simulink model "Control_Unit_Software_Case3"  (R2018b)
settings: Solver=FixedStepAuto  StartTime=0.0  StopTime=2  RelTol=1e-3
values from neighbouring files (symbols this model uses):
  A = [-(bm*(n^2) + bg)/(Jm*(n^2) + Jg) Kt*n/(Jm*(n^2) + Jg) ... (first row only)    [acceptatieTestScript.m]
  B = [0 ... (first row only)    [acceptatieTestScript.m]
  C = [1 0]    [acceptatieTestScript.m]
  D = [0]    [acceptatieTestScript.m]
  Kdi = dlqr(Ad,Bd,Q,R)    [acceptatieTestScript.m]
  n = 16.5    [acceptatieTestScript.m]
  Tsc = 1/20000    (= 5e-05)    [acceptatieTestScript.m]
undefined symbols (not defined in the file or in its folder): DiscIntNeverNeededParam, sigbuilder_block
libraries: dspswit3 x29, simulink x14, powerlib_meascontrol x6, dspsigops x4, pePwmGenerator x4, peLuenbergerObserver x2, peGeneralControl x1
(part 1 of 2)
settings Model: Creator=Roberto  LastModifiedBy=Roberto

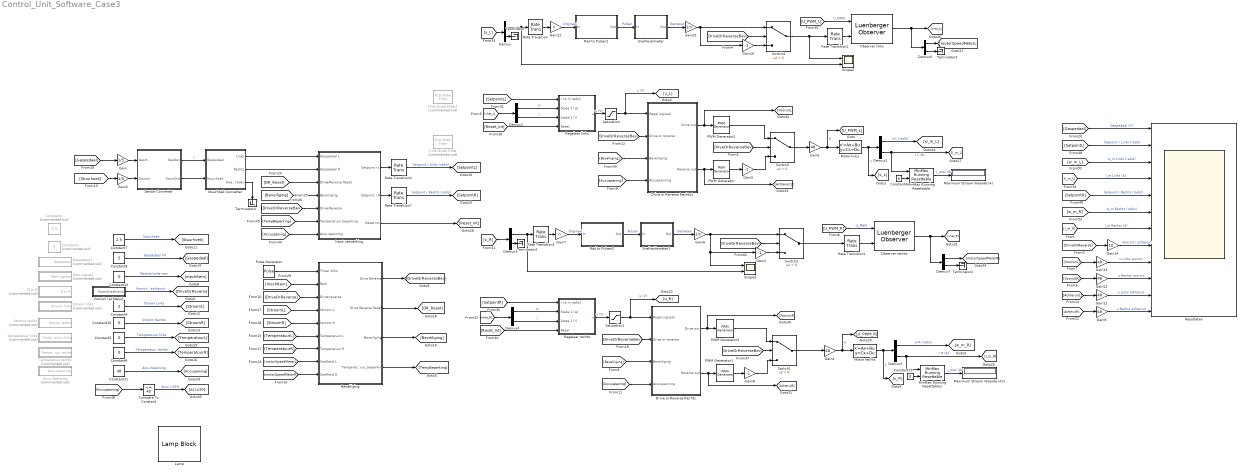
== system Control_Unit_Software_Case3 ==
  Accu Spanning : Subsystem  Tag=STV Subsys  Commented=on  LoadFcn=sigbuilder_block('load');  StartFcn=sigbuilder_block('start');  StopFcn=sigbuilder_block('stop');  ClipboardFcn=sigbuilder_block('clipboard');  mask(Sigbuilder block){tuvar=[0:10]}
      mask help: Simulink:masks:SigbuilderBlock_MD
      mask init:
      | if ~strcmp(get_param(bdroot(gcbh),'SimulationStatus'),'stopped') tuvar = sigbuilder_block('maskInit'); end
      settings: CopyFcn=sigbuilder_block('copy');  DeleteFcn=sigbuilder_block('delete');  ModelCloseFcn=sigbuilder_block('modelClose');  PreSaveFcn=sigbuilder_block('preSave');  PauseFcn=sigbuilder_block('pause');  ContinueFcn=sigbuilder_block('continue');  NameChangeFcn=sigbuilder_block('namechange');  OpenFcn=sigbuilder_block('open',[341.25 138 550.5 359.25 ]);  CloseFcn=sigbuilder_block('close');
      mask Display: plot(0, 0, 100, 100,[2, 2, 32, 32, 2], [68, 8, 8, 68, 68],[32, 2], [38, 38], [32, 19, 2],[53, 60, 44], [32, 17, 17, 2],[16, 16, 31, 31]);txt = getActiveGroup(gcbh);text(2, 100, txt,'verticalAlignment', 'top');
  Beveiliging : Subsystem
  Compare To Constant : simulink/Logic and Bit Operations/Compare To Constant  relop=<=  const=40  OutDataTypeStr=boolean
  Constant{4..6,9..10,13,15} (7 alike) : Constant  Value=0
  Constant11 : Constant  Value=48
  Constant2 : Constant  Commented=on  Value=2.5
  Constant3 : Constant  Commented=on  Value=5
  Constant7 : Constant  Value=2.5
  Constant8 : Constant  Value=5
  D or R : Subsystem  Tag=STV Subsys  Commented=on  LoadFcn=sigbuilder_block('load');  StartFcn=sigbuilder_block('start');  StopFcn=sigbuilder_block('stop');  ClipboardFcn=sigbuilder_block('clipboard');  mask(Sigbuilder block){tuvar=[0:10]}
      mask help: Simulink:masks:SigbuilderBlock_MD
      mask init:
      | if ~strcmp(get_param(bdroot(gcbh),'SimulationStatus'),'stopped') tuvar = sigbuilder_block('maskInit'); end
      settings: CopyFcn=sigbuilder_block('copy');  DeleteFcn=sigbuilder_block('delete');  ModelCloseFcn=sigbuilder_block('modelClose');  PreSaveFcn=sigbuilder_block('preSave');  PauseFcn=sigbuilder_block('pause');  ContinueFcn=sigbuilder_block('continue');  NameChangeFcn=sigbuilder_block('namechange');  OpenFcn=sigbuilder_block('open',[437.6 153 550.4 359.25 ]);  CloseFcn=sigbuilder_block('close');
      mask Display: plot(0, 0, 100, 100,[2, 2, 32, 32, 2], [68, 8, 8, 68, 68],[32, 2], [38, 38], [32, 19, 2],[53, 60, 44], [32, 17, 17, 2],[16, 16, 31, 31]);txt = getActiveGroup(gcbh);text(2, 100, txt,'verticalAlignment', 'top');
  Demux{,1..7} (8 alike) : Demux  Outputs=2
  Drive or Reverse Rechts : Subsystem
  Drive or Reverse Rechts1 : Subsystem
  First-Order Filter : powerlib_meascontrol/Filters/First-Order Filter  Commented=on  FilterType=Lowpass  Tc=1.2  Ts=Tsc  Initialize=on  Vac_Init=[0, 0, 60]  Vdc_Init=0  PlotResponse=off  FreqRange="[0,  200,  1]"
      settings: SourceProductName=Simscape Power Systems
  First-Order Filter1 : powerlib_meascontrol/Filters/First-Order Filter  Commented=on  FilterType=Lowpass  Tc=1.2  Ts=Tsc  Initialize=on  Vac_Init=[0, 0, 60]  Vdc_Init=0  PlotResponse=off  FreqRange="[0,  200,  1]"
      settings: SourceProductName=Simscape Power Systems
  Gain : Gain  Gain=1/5
  Gain{1,4,9,11..13} (6 alike) : Gain  Gain=48
  Gain{2,5,8,10} (4 alike) : Gain  Gain=-1
  Gain14 : Gain  Gain=10
  Gain21 : Gain  Gain=1/n
  Gain22 : Gain  Gain=n
  Gain3 : Gain  Gain=1/5
  Gain6 : Gain  Gain=1/n
  Gain7 : Gain  Gain=n
  Gaspedaal1 : Subsystem  Tag=STV Subsys  Commented=on  LoadFcn=sigbuilder_block('load');  StartFcn=sigbuilder_block('start');  StopFcn=sigbuilder_block('stop');  ClipboardFcn=sigbuilder_block('clipboard');  mask(Sigbuilder block){tuvar=[0:10]}
      mask help: Simulink:masks:SigbuilderBlock_MD
      mask init:
      | if ~strcmp(get_param(bdroot(gcbh),'SimulationStatus'),'stopped') tuvar = sigbuilder_block('maskInit'); end
      settings: CopyFcn=sigbuilder_block('copy');  DeleteFcn=sigbuilder_block('delete');  ModelCloseFcn=sigbuilder_block('modelClose');  PreSaveFcn=sigbuilder_block('preSave');  PauseFcn=sigbuilder_block('pause');  ContinueFcn=sigbuilder_block('continue');  NameChangeFcn=sigbuilder_block('namechange');  OpenFcn=sigbuilder_block('open',[468 234 550.5 278.25 ]);  CloseFcn=sigbuilder_block('close');
      mask Display: plot(0, 0, 100, 100,[2, 2, 32, 32, 2], [68, 8, 8, 68, 68],[32, 2], [38, 38], [32, 19, 2],[53, 60, 44], [32, 17, 17, 2],[16, 16, 31, 31]);txt = getActiveGroup(gcbh);text(2, 100, txt,'verticalAlignment', 'top');
  Input verwerking : Subsystem
  Lamp : LampBlock  WebBlockId=979
  Maximum Stroom Waarde (A) : Display
  Maximum Stroom Waarde (A)1 : Display
  MinMax Running Resettable : simulink/Math Operations/MinMax Running Resettable  Function=max  vinit=0.0
  MinMax Running Resettable1 : simulink/Math Operations/MinMax Running Resettable  Function=max  vinit=0.0
  Motor links : StateSpace  A=A  B=B  C=eye(2)  D=[0; 0]  InitialCondition=0
  Motor rechts : StateSpace  A=A  B=B  C=eye(2)  D=[0; 0]  InitialCondition=0
  Observer links : peLuenbergerObserver/Luenberger Observer  StateSpaceType=Continuous-time  Ad=Adh  Bd=Bdh  Cd=C  Dd=0  A=A  B=B  C=C  D=D  ObserverDesign=Observer gain  Ld=L  DesiredEigenvalues=eigenVal  x0=[0 0]  Tsd=0.1  Ts=1e-6
  Observer rechts : peLuenbergerObserver/Luenberger Observer  StateSpaceType=Continuous-time  Ad=Adh  Bd=Bdh  Cd=C  Dd=0  A=A  B=B  C=C  D=D  ObserverDesign=Observer gain  Ld=L  DesiredEigenvalues=eigenVal  x0=[0 0]  Tsd=0.1  Ts=1e-6
  PWM Generator{,1..3} (4 alike) : pePwmGenerator/PWM Generator  CarrCount=Up  Tper=1/20000  Ts=1e-6
  Pulse Generator : DiscretePulseGenerator  SampleTime=1/2000
  Rad to Pulsen1 : Subsystem
  Rad to Pulsen2 : Subsystem
  Rate Transition : RateTransition  OutPortSampleTime=1/100000
  Rate Transition1 : RateTransition  OutPortSampleTime=1e-6
  Rate Transition2 : RateTransition  OutPortSampleTime=Tsc
  Rate Transition3 : RateTransition  OutPortSampleTime=1/100000
  Rate Transition4 : RateTransition  OutPortSampleTime=1e-6
  Rate Transition7 : RateTransition  OutPortSampleTime=Tsc
  Regelaar links : Subsystem
  Regelaar rechts : Subsystem
  Rem signaal : Subsystem  Tag=STV Subsys  Commented=on  LoadFcn=sigbuilder_block('load');  StartFcn=sigbuilder_block('start');  StopFcn=sigbuilder_block('stop');  ClipboardFcn=sigbuilder_block('clipboard');  mask(Sigbuilder block){tuvar=[0:10]}
      mask help: Simulink:masks:SigbuilderBlock_MD
      mask init:
      | if ~strcmp(get_param(bdroot(gcbh),'SimulationStatus'),'stopped') tuvar = sigbuilder_block('maskInit'); end
      settings: CopyFcn=sigbuilder_block('copy');  DeleteFcn=sigbuilder_block('delete');  ModelCloseFcn=sigbuilder_block('modelClose');  PreSaveFcn=sigbuilder_block('preSave');  PauseFcn=sigbuilder_block('pause');  ContinueFcn=sigbuilder_block('continue');  NameChangeFcn=sigbuilder_block('namechange');  OpenFcn=sigbuilder_block('open',[437.6 153 550.4 359.25 ]);  CloseFcn=sigbuilder_block('close');
      mask Display: plot(0, 0, 100, 100,[2, 2, 32, 32, 2], [68, 8, 8, 68, 68],[32, 2], [38, 38], [32, 19, 2],[53, 60, 44], [32, 17, 17, 2],[16, 16, 31, 31]);txt = getActiveGroup(gcbh);text(2, 100, txt,'verticalAlignment', 'top');
  Resultaten : Scope  NumInputPorts=12
  Saturation : Saturate  UpperLimit=60  LowerLimit=-60
  Saturation1 : Saturate  UpperLimit=60  LowerLimit=-60
  Scope3 : Scope  NumInputPorts=2
  Scope5 : Scope  NumInputPorts=2
  Sensor Converter : Subsystem
  Snelheidsmeter : Subsystem
  Snelheidsmeter1 : Subsystem
  Stroom links : Subsystem  Tag=STV Subsys  Commented=on  LoadFcn=sigbuilder_block('load');  StartFcn=sigbuilder_block('start');  StopFcn=sigbuilder_block('stop');  ClipboardFcn=sigbuilder_block('clipboard');  mask(Sigbuilder block){tuvar=[0:10]}
      mask help: Simulink:masks:SigbuilderBlock_MD
      mask init:
      | if ~strcmp(get_param(bdroot(gcbh),'SimulationStatus'),'stopped') tuvar = sigbuilder_block('maskInit'); end
      settings: CopyFcn=sigbuilder_block('copy');  DeleteFcn=sigbuilder_block('delete');  ModelCloseFcn=sigbuilder_block('modelClose');  PreSaveFcn=sigbuilder_block('preSave');  PauseFcn=sigbuilder_block('pause');  ContinueFcn=sigbuilder_block('continue');  NameChangeFcn=sigbuilder_block('namechange');  OpenFcn=sigbuilder_block('open',[437.6 153 550.4 359.25 ]);  CloseFcn=sigbuilder_block('close');
      mask Display: plot(0, 0, 100, 100,[2, 2, 32, 32, 2], [68, 8, 8, 68, 68],[32, 2], [38, 38], [32, 19, 2],[53, 60, 44], [32, 17, 17, 2],[16, 16, 31, 31]);txt = getActiveGroup(gcbh);text(2, 100, txt,'verticalAlignment', 'top');
  Stroom rechts : Subsystem  Tag=STV Subsys  Commented=on  LoadFcn=sigbuilder_block('load');  StartFcn=sigbuilder_block('start');  StopFcn=sigbuilder_block('stop');  ClipboardFcn=sigbuilder_block('clipboard');  mask(Sigbuilder block){tuvar=[0:10]}
      mask help: Simulink:masks:SigbuilderBlock_MD
      mask init:
      | if ~strcmp(get_param(bdroot(gcbh),'SimulationStatus'),'stopped') tuvar = sigbuilder_block('maskInit'); end
      settings: CopyFcn=sigbuilder_block('copy');  DeleteFcn=sigbuilder_block('delete');  ModelCloseFcn=sigbuilder_block('modelClose');  PreSaveFcn=sigbuilder_block('preSave');  PauseFcn=sigbuilder_block('pause');  ContinueFcn=sigbuilder_block('continue');  NameChangeFcn=sigbuilder_block('namechange');  OpenFcn=sigbuilder_block('open',[437.6 153 550.4 359.25 ]);  CloseFcn=sigbuilder_block('close');
      mask Display: plot(0, 0, 100, 100,[2, 2, 32, 32, 2], [68, 8, 8, 68, 68],[32, 2], [38, 38], [32, 19, 2],[53, 60, 44], [32, 17, 17, 2],[16, 16, 31, 31]);txt = getActiveGroup(gcbh);text(2, 100, txt,'verticalAlignment', 'top');
  Stuurhoek Converter : Subsystem
  Switch{1..4} (4 alike) : Switch  Criteria=u2 > Threshold
  Temperatuur links : Subsystem  Tag=STV Subsys  Commented=on  LoadFcn=sigbuilder_block('load');  StartFcn=sigbuilder_block('start');  StopFcn=sigbuilder_block('stop');  ClipboardFcn=sigbuilder_block('clipboard');  mask(Sigbuilder block){tuvar=[0:10]}
      mask help: Simulink:masks:SigbuilderBlock_MD
      mask init:
      | if ~strcmp(get_param(bdroot(gcbh),'SimulationStatus'),'stopped') tuvar = sigbuilder_block('maskInit'); end
      settings: CopyFcn=sigbuilder_block('copy');  DeleteFcn=sigbuilder_block('delete');  ModelCloseFcn=sigbuilder_block('modelClose');  PreSaveFcn=sigbuilder_block('preSave');  PauseFcn=sigbuilder_block('pause');  ContinueFcn=sigbuilder_block('continue');  NameChangeFcn=sigbuilder_block('namechange');  OpenFcn=sigbuilder_block('open',[437.6 153 550.4 359.25 ]);  CloseFcn=sigbuilder_block('close');
      mask Display: plot(0, 0, 100, 100,[2, 2, 32, 32, 2], [68, 8, 8, 68, 68],[32, 2], [38, 38], [32, 19, 2],[53, 60, 44], [32, 17, 17, 2],[16, 16, 31, 31]);txt = getActiveGroup(gcbh);text(2, 100, txt,'verticalAlignment', 'top');
  Temperatuur rechts : Subsystem  Tag=STV Subsys  Commented=on  LoadFcn=sigbuilder_block('load');  StartFcn=sigbuilder_block('start');  StopFcn=sigbuilder_block('stop');  ClipboardFcn=sigbuilder_block('clipboard');  mask(Sigbuilder block){tuvar=[0:10]}
      mask help: Simulink:masks:SigbuilderBlock_MD
      mask init:
      | if ~strcmp(get_param(bdroot(gcbh),'SimulationStatus'),'stopped') tuvar = sigbuilder_block('maskInit'); end
      settings: CopyFcn=sigbuilder_block('copy');  DeleteFcn=sigbuilder_block('delete');  ModelCloseFcn=sigbuilder_block('modelClose');  PreSaveFcn=sigbuilder_block('preSave');  PauseFcn=sigbuilder_block('pause');  ContinueFcn=sigbuilder_block('continue');  NameChangeFcn=sigbuilder_block('namechange');  OpenFcn=sigbuilder_block('open',[437.6 153 550.4 359.25 ]);  CloseFcn=sigbuilder_block('close');
      mask Display: plot(0, 0, 100, 100,[2, 2, 32, 32, 2], [68, 8, 8, 68, 68],[32, 2], [38, 38], [32, 19, 2],[53, 60, 44], [32, 17, 17, 2],[16, 16, 31, 31]);txt = getActiveGroup(gcbh);text(2, 100, txt,'verticalAlignment', 'top');
  Terminator{,1..4} (5 alike) : Terminator
  Vooruit / achteruit : Subsystem  Tag=STV Subsys  LoadFcn=sigbuilder_block('load');  StartFcn=sigbuilder_block('start');  StopFcn=sigbuilder_block('stop');  ClipboardFcn=sigbuilder_block('clipboard');  mask(Sigbuilder block){tuvar=[0:10]}
      mask help: Simulink:masks:SigbuilderBlock_MD
      mask init:
      | if ~strcmp(get_param(bdroot(gcbh),'SimulationStatus'),'stopped') tuvar = sigbuilder_block('maskInit'); end
      settings: CopyFcn=sigbuilder_block('copy');  DeleteFcn=sigbuilder_block('delete');  ModelCloseFcn=sigbuilder_block('modelClose');  PreSaveFcn=sigbuilder_block('preSave');  PauseFcn=sigbuilder_block('pause');  ContinueFcn=sigbuilder_block('continue');  NameChangeFcn=sigbuilder_block('namechange');  OpenFcn=sigbuilder_block('open',[468 255.75 550.5 237.75 ]);  CloseFcn=sigbuilder_block('close');
      mask Display: plot(0, 0, 100, 100,[2, 2, 32, 32, 2], [68, 8, 8, 68, 68],[32, 2], [38, 38], [32, 19, 2],[53, 60, 44], [32, 17, 17, 2],[16, 16, 31, 31]);txt = getActiveGroup(gcbh);text(2, 100, txt,'verticalAlignment', 'top');
  wires:
  Gain1/1 -> [U_PWM_L], Motor links/1  "U"
  Switch2/1 -> Gain1/1
  Demux1/2 -> Regelaar links/3(State 1 (I))  "I"
  Demux1/1 -> Regelaar links/2(State 1 (w))  "w"
  [Reset_Int] -> Regelaar links/4(Reset)
  [xhat_L] -> Demux1/1
  MinMax Running Resettable/1 -> Maximum Stroom Waarde (A)/1  "I_max (A)"
  Constant4/1 -> MinMax Running Resettable/2
  Demux2/2 -> [I_m_L], MinMax Running Resettable/1  "I L (A)"
  Demux2/1 -> [w_m_L]  "w L (rad/s)"
  Motor links/1 -> Demux2/1, [x_L]  "x"
  [U_PWM_L] -> Observer links/1  "U_PWM"
  Rad to Pulsen1/1(Out) -> Snelheidsmeter/1(In)  "Pulsen"
  Rate Transition1/1 -> Observer links/2
  Rate Transition/1 -> Gain22/1
  Snelheidsmeter/1(Out) -> Gain21/1  "Gemeten"
  Gain22/1 -> Rad to Pulsen1/1(In)  "Orgineel"
  Switch4/1 -> Rate Transition1/1, Scope5/1
  [x_L] -> Demux/1
  Demux/1 -> Scope5/2, Rate Transition/1
  Demux/2 -> Terminator/1
  Observer links/1 -> Demux6/1, [xhat_L]
  Beveiliging/1("Drive Reverse ") -> [DriveOrReverseBev]
  Gain/1 -> Sensor Converter/1(GasIn)
  Stuurhoek Converter/1(Links) -> Input verwerking/1(Gaspedaal L)
  Input verwerking/1(Setpoint r L) -> Rate Transition2/1
  Gain3/1 -> Sensor Converter/2(StuurIn)
  Input verwerking/3(Reset Int) -> [Reset_Int]
  Sensor Converter/2(StuurOut) -> Stuurhoek Converter/2(Stuurhoek)
  [DriveOrReverse] -> Beveiliging/3(Drive/reverse)
  [motorSpeedMeterR] -> Beveiliging/9(Snelheid R)
  [TemperatuurL] -> Beveiliging/6(Temperatuur L)
  [StroomR] -> Beveiliging/5(Stroom R)
  [StroomL] -> Beveiliging/4(Stroom L)
  Beveiliging/3(Beveiliging) -> [Beveiliging]
  [motorSpeedMeterL] -> Beveiliging/8(Snelheid L)
  Input verwerking/2(Setpoint r R) -> Rate Transition7/1
  Beveiliging/2(Drive Reverse Reset) -> [DR_Reset]
  [Stuurhoek] -> Gain3/1
  Stuurhoek Converter/2(Rechts) -> Input verwerking/2(Gaspedaal R)
  [mechRem] -> Beveiliging/2(Rem)
  [DR_Reset] -> Input verwerking/3(Drive/Reverse Reset)
  [Beveiliging] -> Input verwerking/4(Beveiliging)
  Pulse Generator/1 -> Beveiliging/1(Timer 1khz)
  [Gaspedaal] -> Gain/1
  [DriveOrReverseBev] -> Input verwerking/5(Drive/Reverse)
  Rate Transition7/1 -> [SetpointR]  "Setpoint r Rechts (rad/s)"
  Rate Transition2/1 -> [SetpointL]  "Setpoint r Links (rad/s)"
  [TemperatuurR] -> Beveiliging/7(Temperatuur R)
  Observer rechts/1 -> Demux7/1, [xhat_R]
  Demux5/1 -> [w_m_R]  "w R (rad/s)"
  Demux4/2 -> Regelaar rechts/3(State 1 (I))  "I"
  Rate Transition4/1 -> Observer rechts/2
  Gain7/1 -> Rad to Pulsen2/1(In)  "Orgineel"
  Switch1/1 -> Gain4/1
  [U_PWM_R] -> Observer rechts/1  "U_PWM"
  Snelheidsmeter1/1(Out) -> Gain6/1  "Gemeten"
  [Reset_Int] -> Regelaar rechts/4(Reset)
  [xhat_R] -> Demux4/1
  Demux3/1 -> Scope3/2, Rate Transition3/1
  MinMax Running Resettable1/1 -> Maximum Stroom Waarde (A)1/1  "I_max (A)"
  Demux5/2 -> [I_m_R], MinMax Running Resettable1/1  "I R (A)"
  [x_R] -> Demux3/1
  Motor rechts/1 -> [x_R], Demux5/1  "x"
  Rad to Pulsen2/1(Out) -> Snelheidsmeter1/1(In)  "Pulsen"
  Demux4/1 -> Regelaar rechts/2(State 1 (w))  "w"
  Constant15/1 -> MinMax Running Resettable1/2
  Gain4/1 -> [U_PWM_R], Motor rechts/1  "U"
  Demux3/2 -> Terminator2/1
  Rate Transition3/1 -> Gain7/1
  [SetpointL] -> Regelaar links/1(r (w in rad/s))
  [SetpointR] -> Regelaar rechts/1(r (w in rad/s))
  [Beveiliging] -> Drive or Reverse Rechts/3(Beveiliging)
  [DriveOrReverseBev] -> Switch1/2
  Drive or Reverse Rechts/1(Drive out) -> [VooruitR], PWM Generator3/1
  [Accuspaning] -> Drive or Reverse Rechts/4(Accuspanning)
  [DriveOrReverseBev] -> Drive or Reverse Rechts/2(Drive or reverse)
  Drive or Reverse Rechts/2(Reverse out) -> [AchteruitR], PWM Generator1/1
  Regelaar rechts/1(u) -> Saturation1/1  "u (V)"
  [Beveiliging] -> Drive or Reverse Rechts1/3(Beveiliging)
  [DriveOrReverseBev] -> Switch2/2
  Drive or Reverse Rechts1/1(Drive out) -> [VooruitL], PWM Generator2/1
  [Accuspaning] -> Drive or Reverse Rechts1/4(Accuspanning)
  [DriveOrReverseBev] -> Drive or Reverse Rechts1/2(Drive or reverse)
  Drive or Reverse Rechts1/2(Reverse out) -> [AchteruitL], PWM Generator/1
  Regelaar links/1(u) -> Saturation/1  "u (V)"
  Constant8/1 -> [Gaspedaal]  "Gaspedaal (V)"
  Constant13/1 -> [mechRem]  "Mechanische rem"
  Vooruit / achteruit/1(Vooruit/achteruit) -> [DriveOrReverse]  "Vooruit / achteruit"
  Constant9/1 -> [StroomL]  "Stroom Links"
  Constant6/1 -> [TemperatuurR]  "Temperatuur rechts"
  Constant7/1 -> [Stuurhoek]  "Stuurhoek"
  Constant10/1 -> [StroomR]  "Stroom Rechts"
  Constant5/1 -> [TemperatuurL]  "Temperatuur links"
  Constant11/1 -> [Accuspaning]  "Accu Spanning"
  Beveiliging/4(Temperatuur_beperking) -> [TempBeperking]
  [Accuspaning] -> Input verwerking/7(Accu spanning)
  [TempBeperking] -> Input verwerking/6(Temperatuur beperking)
  Gain6/1 -> Scope3/1, Gain2/1, Switch3/1
  [DriveOrReverseBev] -> Switch3/2
  Gain2/1 -> Switch3/3
  Switch3/1 -> Rate Transition4/1
  Gain21/1 -> Gain10/1, Switch4/1
  Gain10/1 -> Switch4/3
  [DriveOrReverseBev] -> Switch4/2
  Gain5/1 -> Switch2/3
  Gain8/1 -> Switch1/3
  PWM Generator/1 -> Gain5/1
  PWM Generator2/1 -> Switch2/1
  PWM Generator1/1 -> Gain8/1
  PWM Generator3/1 -> Switch1/1
  Saturation/1 -> [u_L], Drive or Reverse Rechts1/1(Regel signaal)  "u (V)"
  Saturation1/1 -> [u_R], Drive or Reverse Rechts/1(Regel signaal)  "u (V)"
  Demux6/1 -> [motorSpeedMeterL]
  Demux7/1 -> [motorSpeedMeterR]
  Demux7/2 -> Terminator1/1
  Demux6/2 -> Terminator3/1
  Compare To Constant/1 -> [accu10]  "Accu <10%"
  [Accuspaning] -> Compare To Constant/1
  Sensor Converter/1(GasOut) -> Stuurhoek Converter/1("Gaspedaal ")  "r"
  [Gaspedaal] -> Resultaten/1  "Gaspedaal (V)"
  [SetpointR] -> Resultaten/5  "Setpoint r Rechts (rad/s)"
  [w_m_L] -> Resultaten/3  "w_m Links (rad/s)"
  [SetpointL] -> Resultaten/2  "Setpoint r Links (rad/s)"
  [w_m_R] -> Resultaten/6  "w_m Rechts (rad/s)"
  [DriveOrReverse] -> Gain14/1
  [VooruitL] -> Gain13/1
  [VooruitR] -> Gain12/1
  [AchteruitL] -> Gain11/1
  [AchteruitR] -> Gain9/1
  Gain9/1 -> Resultaten/12  "u Rechts achteruit"
  Gain11/1 -> Resultaten/11  "u Links achteruit"
  Gain12/1 -> Resultaten/10  "u Rechts vooruit"
  Gain13/1 -> Resultaten/9  "u Links vooruit"
  Gain14/1 -> Resultaten/8  "Vooruit / achteruit"
  Stuurhoek Converter/3(Hoek in graden) -> Terminator4/1
  [I_m_L] -> Resultaten/4  "I_m Links (A)"
  [I_m_R] -> Resultaten/7  "I_m Rechts (A)"

== system Control_Unit_Software_Case3/Accu Spanning ==
  Demux : Demux  Tag=STV Demux  Outputs=1
  FromWs : FromWorkspace  Tag=STV FromWs  VariableName=tuvar  SampleTime=0
      SigBuilderData=|
      | common.afterFinalStr = 'Extrapolate'
      | common.sampleTime = 0
      | dataSet.timeRange = [0 20]
      | dataSet.name = 'Group 1'
      | sbobj.Groups.Name = 'Group 1'
      | sbobj.Groups.Signals.Name = 'Accu spanning'
      | sbobj.Groups.Signals.XData = [0 5 10 14.65 16.1 17.75 20]
      | sbobj.Groups.Signals.YData = [48 60 48 40 30 48 48]
      | sbobj.Groups.TimeRange = [0 20]
  Accu spanning : Outport  Tag=STV Outport
  wires:
  Demux/1 -> Accu spanning/1
  FromWs/1 -> Demux/1

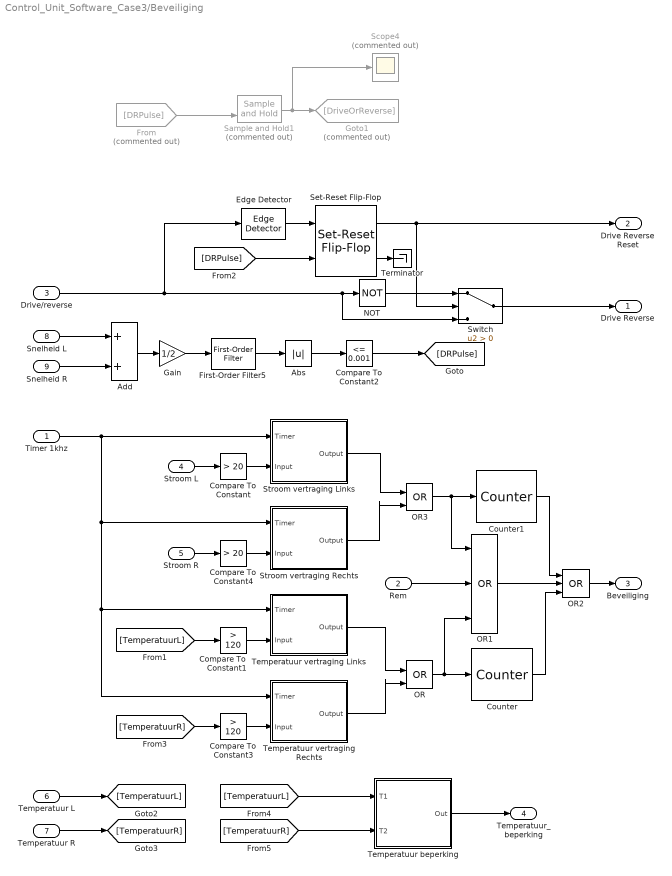
== system Control_Unit_Software_Case3/Beveiliging ==
  Timer 1khz : Inport
  Rem : Inport  Port=2
  Drive/reverse : Inport  Port=3
  Stroom L : Inport  Port=4
  Stroom R : Inport  Port=5
  Temperatuur L : Inport  Port=6
  Temperatuur R : Inport  Port=7
  Snelheid L : Inport  Port=8
  Snelheid R : Inport  Port=9
  Abs : Abs
  Add : Sum
  Compare To Constant : simulink/Logic and Bit Operations/Compare To Constant  relop=>  const=20  OutDataTypeStr=boolean
  Compare To Constant1 : simulink/Logic and Bit Operations/Compare To Constant  relop=>  const=120  OutDataTypeStr=boolean
  Compare To Constant2 : simulink/Logic and Bit Operations/Compare To Constant  relop=<=  const=0.001  OutDataTypeStr=boolean
  Compare To Constant3 : simulink/Logic and Bit Operations/Compare To Constant  relop=>  const=120  OutDataTypeStr=boolean
  Compare To Constant4 : simulink/Logic and Bit Operations/Compare To Constant  relop=>  const=20  OutDataTypeStr=boolean
  Counter : dspswit3/Counter  Direction=Up  CountEvent=Rising edge  CounterSize=32 bits  MaxCount=255  InitialCount=0  Output=Hit  HitValue=3  ResetInput=off  SamplesPerFrame=1  Ts=1  CntDtype=double  HitDtype=Logical
  Counter1 : dspswit3/Counter  Direction=Up  CountEvent=Rising edge  CounterSize=32 bits  MaxCount=255  InitialCount=0  Output=Hit  HitValue=3  ResetInput=off  SamplesPerFrame=1  Ts=1  CntDtype=double  HitDtype=Logical
  Edge Detector : powerlib_meascontrol/Logic/Edge Detector  model=Either  ic=0  Ts=-1
      settings: SourceProductName=Simscape Power Systems  SourceProductBaseCode=PS
  First-Order Filter5 : powerlib_meascontrol/Filters/First-Order Filter  FilterType=Lowpass  Tc=10e-3  Ts=Tsc  Initialize=on  Vac_Init=[0, 0, 50]  Vdc_Init=0  PlotResponse=off  FreqRange="[0,  200,  1]"
      settings: SourceProductName=Simscape Power Systems
  From : From  Commented=on  GotoTag=DRPulse
  Gain : Gain  Gain=1/2
  Goto1 : Goto  Commented=on  GotoTag=DriveOrReverse
  NOT : Logic  Operator=NOT  IconShape=distinctive  AllPortsSameDT=off  OutDataTypeStr=boolean
  OR : Logic  Operator=OR  IconShape=distinctive  AllPortsSameDT=off  OutDataTypeStr=boolean
  OR1 : Logic  Operator=OR  Inputs=3  IconShape=distinctive  AllPortsSameDT=off  OutDataTypeStr=boolean
  OR2 : Logic  Operator=OR  Inputs=3  IconShape=distinctive  AllPortsSameDT=off  OutDataTypeStr=boolean
  OR3 : Logic  Operator=OR  IconShape=distinctive  AllPortsSameDT=off  OutDataTypeStr=boolean
  Sample and Hold1 : powerlib_meascontrol/Additional Components/Sample and Hold  Commented=on  ic=0  Ts=0
      settings: SourceProductName=Simscape Power Systems  SourceProductBaseCode=PS
  Scope4 : Scope  Commented=on
  Set-Reset Flip-Flop : peGeneralControl/Set-Reset Flip-Flop  LabelModeActiveChoice=Discrete  UndefState=Set  Q0=0  Ts=-1
  Stroom vertraging Links : Subsystem
  Stroom vertraging Rechts : Subsystem
  Switch : Switch  Criteria=u2 > Threshold
  Temperatuur beperking : Subsystem
  Temperatuur vertraging Links : Subsystem
  "Temperatuur vertraging Rechts " : Subsystem
  Terminator : Terminator
  "Drive Reverse " : Outport
  Drive Reverse Reset : Outport  Port=2
  Beveiliging : Outport  Port=3
  Temperatuur_beperking : Outport  Port=4
  wires:
  Stroom L/1 -> Compare To Constant/1
  Compare To Constant1/1 -> Temperatuur vertraging Links/2(Input)
  Edge Detector/1 -> Set-Reset Flip-Flop/1
  Set-Reset Flip-Flop/1 -> Switch/2, Drive Reverse Reset/1
  Sample and Hold1/1 -> Scope4/1, Goto1/1
  Abs/1 -> Compare To Constant2/1
  Compare To Constant2/1 -> [DRPulse]
  [DRPulse] -> Set-Reset Flip-Flop/2
  Drive/reverse/1 -> Edge Detector/1, Switch/3, NOT/1
  From/1 -> Sample and Hold1/2
  Snelheid L/1 -> Add/1
  Snelheid R/1 -> Add/2
  Add/1 -> Gain/1
  Gain/1 -> First-Order Filter5/1
  Compare To Constant3/1 -> "Temperatuur vertraging Rechts "/2(Input)
  Timer 1khz/1 -> Stroom vertraging Rechts/1(Timer), Temperatuur vertraging Links/1(Timer), "Temperatuur vertraging Rechts "/1(Timer), Stroom vertraging Links/1(Timer)
  Compare To Constant4/1 -> Stroom vertraging Rechts/2(Input)
  Stroom R/1 -> Compare To Constant4/1
  Rem/1 -> OR1/2
  Switch/1 -> "Drive Reverse "/1
  NOT/1 -> Switch/1
  OR/1 -> OR1/3, Counter/1
  Temperatuur vertraging Links/1(Output) -> OR/1
  "Temperatuur vertraging Rechts "/1(Output) -> OR/2
  OR2/1 -> Beveiliging/1
  Counter/1 -> OR2/3
  OR1/1 -> OR2/2
  Set-Reset Flip-Flop/2 -> Terminator/1
  First-Order Filter5/1 -> Abs/1
  Temperatuur L/1 -> [TemperatuurL]
  Temperatuur R/1 -> [TemperatuurR]
  [TemperatuurL] -> Compare To Constant1/1
  [TemperatuurR] -> Compare To Constant3/1
  [TemperatuurL] -> Temperatuur beperking/1(T1)
  [TemperatuurR] -> Temperatuur beperking/2(T2)
  Temperatuur beperking/1(Out) -> Temperatuur_beperking/1
  Compare To Constant/1 -> Stroom vertraging Links/2(Input)
  Stroom vertraging Links/1(Output) -> OR3/1
  Stroom vertraging Rechts/1(Output) -> OR3/2
  OR3/1 -> Counter1/1, OR1/1
  Counter1/1 -> OR2/1

== system Control_Unit_Software_Case3/D or R ==
  Demux : Demux  Tag=STV Demux  Outputs=1
  FromWs : FromWorkspace  Tag=STV FromWs  VariableName=tuvar  SampleTime=0
      SigBuilderData=|
      | common.afterFinalStr = 'Extrapolate'
      | common.sampleTime = 0
      | dataSet.timeRange = [0 10]
      | dataSet.name = 'Group 1'
      | sbobj.Groups.Name = 'Group 1'
      | sbobj.Groups.Signals.Name = 'D or R'
      | sbobj.Groups.Signals.XData = [0 2 4 4 9 9 10]
      | sbobj.Groups.Signals.YData = [0 0 0 1 1 0 0]
  D or R : Outport  Tag=STV Outport
  wires:
  Demux/1 -> D or R/1
  FromWs/1 -> Demux/1

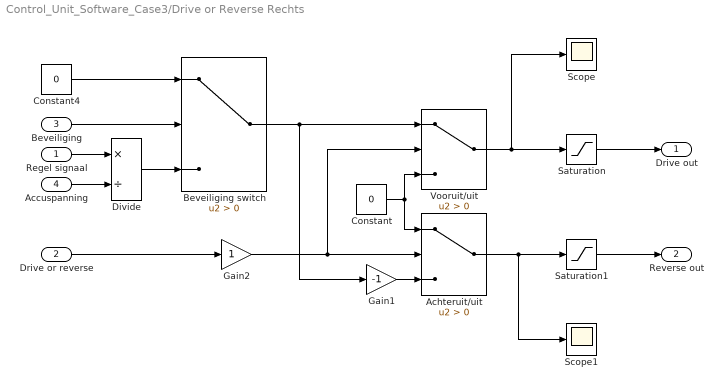
== system Control_Unit_Software_Case3/Drive or Reverse Rechts ==
  Regel signaal : Inport
  Drive or reverse : Inport  Port=2
  Beveiliging : Inport  Port=3
  Accuspanning : Inport  Port=4
  Achteruit/uit : Switch  Criteria=u2 > Threshold
  Beveiliging switch : Switch  Criteria=u2 > Threshold
  Constant : Constant  Value=0
  Constant4 : Constant  Value=0
  Divide : Product  Inputs=*/
  Gain1 : Gain  Gain=-1
  Gain2 : Gain
  Saturation : Saturate  UpperLimit=1  LowerLimit=0
  Saturation1 : Saturate  UpperLimit=1  LowerLimit=0
  Scope : Scope
  Scope1 : Scope
  Vooruit/uit : Switch  Criteria=u2 > Threshold
  Drive out : Outport
  Reverse out : Outport  Port=2
  wires:
  Gain1/1 -> Achteruit/uit/3
  Constant4/1 -> Beveiliging switch/1
  Constant/1 -> Achteruit/uit/1, Vooruit/uit/3
  Beveiliging switch/1 -> Gain1/1, Vooruit/uit/1
  Beveiliging/1 -> Beveiliging switch/2
  Achteruit/uit/1 -> Saturation1/1, Scope1/1
  Gain2/1 -> Vooruit/uit/2, Achteruit/uit/2
  Drive or reverse/1 -> Gain2/1
  Vooruit/uit/1 -> Saturation/1, Scope/1
  Accuspanning/1 -> Divide/2
  Divide/1 -> Beveiliging switch/3
  Regel signaal/1 -> Divide/1
  Saturation/1 -> Drive out/1
  Saturation1/1 -> Reverse out/1

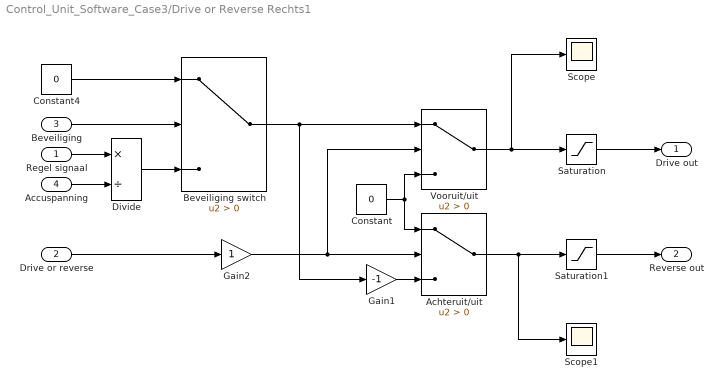
== system Control_Unit_Software_Case3/Drive or Reverse Rechts1 ==
  Regel signaal : Inport
  Drive or reverse : Inport  Port=2
  Beveiliging : Inport  Port=3
  Accuspanning : Inport  Port=4
  Achteruit/uit : Switch  Criteria=u2 > Threshold
  Beveiliging switch : Switch  Criteria=u2 > Threshold
  Constant : Constant  Value=0
  Constant4 : Constant  Value=0
  Divide : Product  Inputs=*/
  Gain1 : Gain  Gain=-1
  Gain2 : Gain
  Saturation : Saturate  UpperLimit=1  LowerLimit=0
  Saturation1 : Saturate  UpperLimit=1  LowerLimit=0
  Scope : Scope
  Scope1 : Scope
  Vooruit/uit : Switch  Criteria=u2 > Threshold
  Drive out : Outport
  Reverse out : Outport  Port=2
  wires:
  Gain1/1 -> Achteruit/uit/3
  Constant4/1 -> Beveiliging switch/1
  Constant/1 -> Achteruit/uit/1, Vooruit/uit/3
  Beveiliging switch/1 -> Gain1/1, Vooruit/uit/1
  Beveiliging/1 -> Beveiliging switch/2
  Achteruit/uit/1 -> Saturation1/1, Scope1/1
  Gain2/1 -> Vooruit/uit/2, Achteruit/uit/2
  Drive or reverse/1 -> Gain2/1
  Vooruit/uit/1 -> Saturation/1, Scope/1
  Accuspanning/1 -> Divide/2
  Divide/1 -> Beveiliging switch/3
  Regel signaal/1 -> Divide/1
  Saturation/1 -> Drive out/1
  Saturation1/1 -> Reverse out/1

== system Control_Unit_Software_Case3/Gaspedaal1 ==
  Demux : Demux  Tag=STV Demux  Outputs=1
  FromWs : FromWorkspace  Tag=STV FromWs  VariableName=tuvar  SampleTime=0
      SigBuilderData=|
      | common.afterFinalStr = 'Extrapolate'
      | common.sampleTime = 0
      | dataSet.timeRange = [0 10]
      | dataSet.name = 'Group 1'
      | sbobj.Groups.Name = 'Group 1'
      | sbobj.Groups.Signals.Name = 'Gaspedaal'
      | sbobj.Groups.Signals.XData = [0 2 10]
      | sbobj.Groups.Signals.YData = [0 5 5]
  Gaspedaal : Outport  Tag=STV Outport
  wires:
  Demux/1 -> Gaspedaal/1
  FromWs/1 -> Demux/1

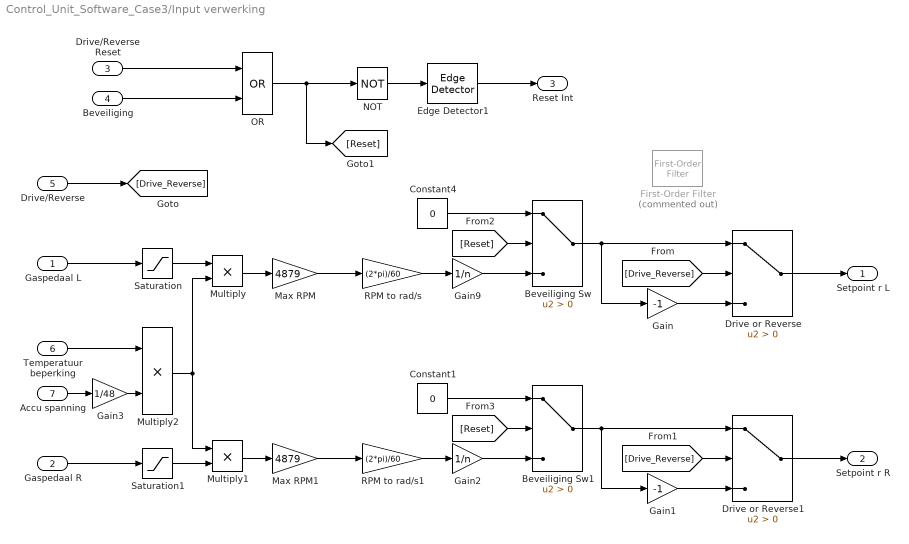
== system Control_Unit_Software_Case3/Input verwerking ==
  Gaspedaal L : Inport
  Gaspedaal R : Inport  Port=2
  Drive/Reverse Reset : Inport  Port=3
  Beveiliging : Inport  Port=4
  Drive/Reverse : Inport  Port=5
  Temperatuur beperking : Inport  Port=6
  Accu spanning : Inport  Port=7
  Beveiliging Sw : Switch  Criteria=u2 > Threshold
  Beveiliging Sw1 : Switch  Criteria=u2 > Threshold
  Constant1 : Constant  Value=0
  Constant4 : Constant  Value=0
  Drive or Reverse : Switch  Criteria=u2 > Threshold
  Drive or Reverse1 : Switch  Criteria=u2 > Threshold
  Edge Detector1 : dspswit3/Edge Detector  InputProcessing=Columns as channels (frame based)
      settings: SourceProductName=DSP System Toolbox  SourceProductBaseCode=DS
  First-Order Filter : powerlib_meascontrol/Filters/First-Order Filter  Commented=on  FilterType=Lowpass  Tc=10e-2  Ts=0  Initialize=on  Vac_Init=[0, 0, 60]  Vdc_Init=0  PlotResponse=off  FreqRange="[0,  200,  1]"
      settings: SourceProductName=Simscape Power Systems
  Gain : Gain  Gain=-1
  Gain1 : Gain  Gain=-1
  Gain2 : Gain  Gain=1/n
  Gain3 : Gain  Gain=1/48
  Gain9 : Gain  Gain=1/n
  Max RPM : Gain  Gain=4879
  Max RPM1 : Gain  Gain=4879
  Multiply : Product
  Multiply1 : Product
  Multiply2 : Product
  NOT : Logic  Operator=NOT  IconShape=distinctive  AllPortsSameDT=off  OutDataTypeStr=boolean
  OR : Logic  Operator=OR  IconShape=distinctive  AllPortsSameDT=off  OutDataTypeStr=boolean
  RPM to rad/s : Gain  Gain=(2*pi)/60
  RPM to rad/s1 : Gain  Gain=(2*pi)/60
  Saturation : Saturate  UpperLimit=1  LowerLimit=0
  Saturation1 : Saturate  UpperLimit=1  LowerLimit=0
  Setpoint r L : Outport
  Setpoint r R : Outport  Port=2
  Reset Int : Outport  Port=3
  wires:
  Constant4/1 -> Beveiliging Sw/1
  Max RPM/1 -> RPM to rad/s/1
  RPM to rad/s/1 -> Gain9/1
  Gaspedaal L/1 -> Saturation/1
  OR/1 -> [Reset], NOT/1
  Gain9/1 -> Beveiliging Sw/3
  Beveiliging Sw/1 -> Gain/1, Drive or Reverse/1
  Gain/1 -> Drive or Reverse/3
  [Drive_Reverse] -> Drive or Reverse/2
  Drive or Reverse/1 -> Setpoint r L/1
  Edge Detector1/1 -> Reset Int/1
  NOT/1 -> Edge Detector1/1
  Beveiliging/1 -> OR/2
  Drive/Reverse Reset/1 -> OR/1
  Max RPM1/1 -> RPM to rad/s1/1
  RPM to rad/s1/1 -> Gain2/1
  Drive or Reverse1/1 -> Setpoint r R/1
  Gaspedaal R/1 -> Saturation1/1
  Gain1/1 -> Drive or Reverse1/3
  Beveiliging Sw1/1 -> Gain1/1, Drive or Reverse1/1
  Constant1/1 -> Beveiliging Sw1/1
  [Drive_Reverse] -> Drive or Reverse1/2
  Gain2/1 -> Beveiliging Sw1/3
  Drive/Reverse/1 -> [Drive_Reverse]
  [Reset] -> Beveiliging Sw/2
  [Reset] -> Beveiliging Sw1/2
  Multiply/1 -> Max RPM/1
  Multiply1/1 -> Max RPM1/1
  Saturation1/1 -> Multiply1/2
  Saturation/1 -> Multiply/1
  Multiply2/1 -> Multiply/2, Multiply1/1
  Temperatuur beperking/1 -> Multiply2/1
  Accu spanning/1 -> Gain3/1
  Gain3/1 -> Multiply2/2

== system Control_Unit_Software_Case3/Rad to Pulsen1 ==
  In : Inport
  Abs2 : Abs
  Compare To Constant1 : simulink/Logic and Bit Operations/Compare To Constant  relop=<=  const=0.5  OutDataTypeStr=boolean
  Discrete-Time Integrator : DiscreteIntegrator  SampleTime=-1  ICPrevOutput=DiscIntNeverNeededParam  ICPrevScaledInput=DiscIntNeverNeededParam
  Gain : Gain  Gain=500/(2*pi)
  Rounding Function : Rounding
  Sum1 : Sum  Inputs=|+-
  Out : Outport
  wires:
  Rounding Function/1 -> Sum1/2
  Discrete-Time Integrator/1 -> Rounding Function/1, Sum1/1
  Compare To Constant1/1 -> Out/1
  Sum1/1 -> Compare To Constant1/1
  Gain/1 -> Discrete-Time Integrator/1
  In/1 -> Abs2/1
  Abs2/1 -> Gain/1

== system Control_Unit_Software_Case3/Rad to Pulsen2 ==
  In : Inport
  Abs2 : Abs
  Compare To Constant1 : simulink/Logic and Bit Operations/Compare To Constant  relop=<=  const=0.5  OutDataTypeStr=boolean
  Discrete-Time Integrator : DiscreteIntegrator  SampleTime=-1  ICPrevOutput=DiscIntNeverNeededParam  ICPrevScaledInput=DiscIntNeverNeededParam
  Gain : Gain  Gain=500/(2*pi)
  Rounding Function : Rounding
  Sum1 : Sum  Inputs=|+-
  Out : Outport
  wires:
  Rounding Function/1 -> Sum1/2
  Discrete-Time Integrator/1 -> Rounding Function/1, Sum1/1
  Compare To Constant1/1 -> Out/1
  Sum1/1 -> Compare To Constant1/1
  Gain/1 -> Discrete-Time Integrator/1
  In/1 -> Abs2/1
  Abs2/1 -> Gain/1

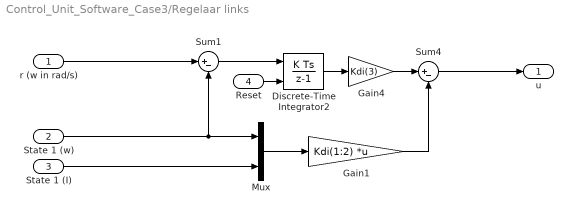
== system Control_Unit_Software_Case3/Regelaar links ==
  r (w in rad/s) : Inport
  State 1 (w) : Inport  Port=2
  State 1 (I) : Inport  Port=3
  Reset : Inport  Port=4
  Discrete-Time Integrator2 : DiscreteIntegrator  gainval=1  ExternalReset=rising  SampleTime=Tsc  ICPrevOutput=DiscIntNeverNeededParam  ICPrevScaledInput=DiscIntNeverNeededParam
  Gain1 : Gain  Gain=Kdi(1:2)  Multiplication=Matrix(K*u)
  Gain4 : Gain  Gain=Kdi(3)
  Mux : Mux  Inputs=2
  Sum1 : Sum  Inputs=|+-
  Sum4 : Sum  Inputs=|+-
  u : Outport
  wires:
  r (w in rad/s)/1 -> Sum1/1
  State 1 (I)/1 -> Mux/2
  Mux/1 -> Gain1/1
  Gain1/1 -> Sum4/2
  Gain4/1 -> Sum4/1
  Sum4/1 -> u/1
  State 1 (w)/1 -> Mux/1, Sum1/2
  Sum1/1 -> Discrete-Time Integrator2/1
  Discrete-Time Integrator2/1 -> Gain4/1
  Reset/1 -> Discrete-Time Integrator2/2

== system Control_Unit_Software_Case3/Regelaar rechts ==
  r (w in rad/s) : Inport
  State 1 (w) : Inport  Port=2
  State 1 (I) : Inport  Port=3
  Reset : Inport  Port=4
  Discrete-Time Integrator2 : DiscreteIntegrator  gainval=1  ExternalReset=rising  SampleTime=Tsc  ICPrevOutput=DiscIntNeverNeededParam  ICPrevScaledInput=DiscIntNeverNeededParam
  Gain1 : Gain  Gain=Kdi(1:2)  Multiplication=Matrix(K*u)
  Gain4 : Gain  Gain=Kdi(3)
  Mux : Mux  Inputs=2
  Sum1 : Sum  Inputs=|+-
  Sum4 : Sum  Inputs=|+-
  u : Outport
  wires:
  r (w in rad/s)/1 -> Sum1/1
  State 1 (I)/1 -> Mux/2
  Mux/1 -> Gain1/1
  Gain1/1 -> Sum4/2
  Gain4/1 -> Sum4/1
  Sum4/1 -> u/1
  State 1 (w)/1 -> Mux/1, Sum1/2
  Sum1/1 -> Discrete-Time Integrator2/1
  Discrete-Time Integrator2/1 -> Gain4/1
  Reset/1 -> Discrete-Time Integrator2/2

== system Control_Unit_Software_Case3/Rem signaal ==
  Demux : Demux  Tag=STV Demux  Outputs=1
  FromWs : FromWorkspace  Tag=STV FromWs  VariableName=tuvar  SampleTime=0
      SigBuilderData=|
      | common.afterFinalStr = 'Extrapolate'
      | common.sampleTime = 0
      | dataSet.timeRange = [0 10]
      | dataSet.name = 'Group 1'
      | sbobj.Groups.Name = 'Group 1'
      | sbobj.Groups.Signals.Name = 'Rem signaal'
      | sbobj.Groups.Signals.XData = [0 6 6 7 7 9 9.6 10]
      | sbobj.Groups.Signals.YData = [0 0 1 1 0 0 0 0]
  Rem signaal : Outport  Tag=STV Outport
  wires:
  Demux/1 -> Rem signaal/1
  FromWs/1 -> Demux/1

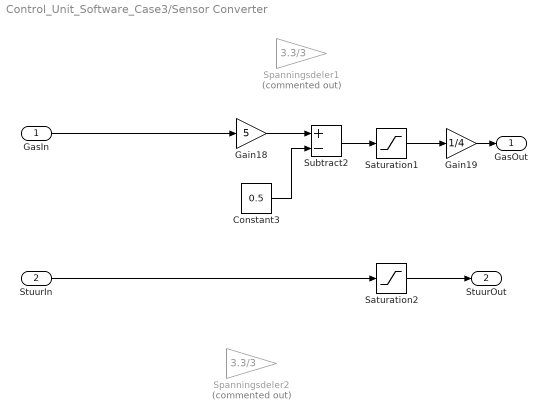
== system Control_Unit_Software_Case3/Sensor Converter ==
  GasIn : Inport
  StuurIn : Inport  Port=2
  Constant3 : Constant  Value=0.5
  Gain18 : Gain  Gain=5
  Gain19 : Gain  Gain=1/4
  Saturation1 : Saturate  UpperLimit=4  LowerLimit=0
  Saturation2 : Saturate  UpperLimit=1  LowerLimit=0
  Spanningsdeler1 : Gain  Commented=on  Gain=3.3/3
  Spanningsdeler2 : Gain  Commented=on  Gain=3.3/3
  Subtract2 : Sum  Inputs=+-
  GasOut : Outport
  StuurOut : Outport  Port=2
  wires:
  Constant3/1 -> Subtract2/2
  Saturation1/1 -> Gain19/1
  GasIn/1 -> Gain18/1
  Gain18/1 -> Subtract2/1
  Gain19/1 -> GasOut/1
  Subtract2/1 -> Saturation1/1
  Saturation2/1 -> StuurOut/1
  StuurIn/1 -> Saturation2/1

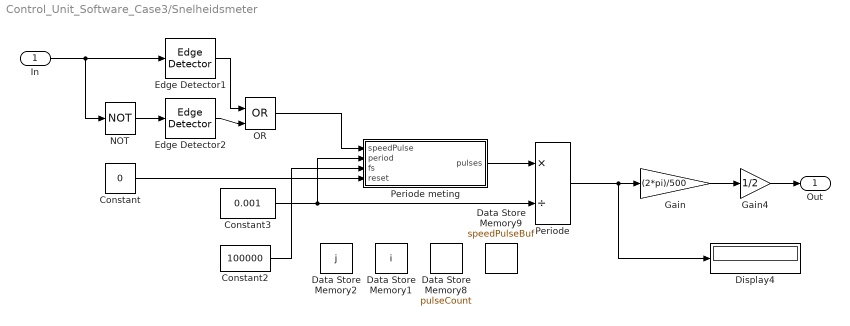
== system Control_Unit_Software_Case3/Snelheidsmeter ==
  In : Inport
  Constant : Constant  Value=0
  Constant2 : Constant  Value=100000
  Constant3 : Constant  Value=0.001
  Data Store Memory1 : DataStoreMemory  DataStoreName=i  ReadBeforeWriteMsg=warning  WriteAfterWriteMsg=warning  WriteAfterReadMsg=warning  InitialValue=1  ShowAdditionalParam=off  OutDataTypeStr=uint32
  Data Store Memory2 : DataStoreMemory  DataStoreName=j  ReadBeforeWriteMsg=warning  WriteAfterWriteMsg=warning  WriteAfterReadMsg=warning  InitialValue=2  ShowAdditionalParam=off  OutDataTypeStr=uint32
  Data Store Memory8 : DataStoreMemory  DataStoreName=pulseCount  ReadBeforeWriteMsg=warning  WriteAfterWriteMsg=warning  WriteAfterReadMsg=warning  ShowAdditionalParam=off  OutDataTypeStr=uint32
  Data Store Memory9 : DataStoreMemory  DataStoreName=speedPulseBuf  ReadBeforeWriteMsg=warning  WriteAfterWriteMsg=warning  WriteAfterReadMsg=warning  ShowAdditionalParam=off  OutDataTypeStr=uint8  Dimensions=10001
  Display4 : Display
  Edge Detector1 : dspswit3/Edge Detector  InputProcessing=Columns as channels (frame based)
      settings: SourceProductName=DSP System Toolbox  SourceProductBaseCode=DS
  Edge Detector2 : dspswit3/Edge Detector  InputProcessing=Columns as channels (frame based)
      settings: SourceProductName=DSP System Toolbox  SourceProductBaseCode=DS
  Gain : Gain  Gain=(2*pi)/500
  Gain4 : Gain  Gain=1/2
  NOT : Logic  Operator=NOT  IconShape=distinctive  AllPortsSameDT=off  OutDataTypeStr=boolean
  OR : Logic  Operator=OR  IconShape=distinctive  AllPortsSameDT=off  OutDataTypeStr=boolean
  Periode : Product  Inputs=*/
  Periode meting : MATLAB Function  TreatAsAtomicUnit=on
  Out : Outport
  wires:
  Constant3/1 -> Periode/2, Periode meting/2(period)
  Periode/1 -> Gain/1, Display4/1
  Constant2/1 -> Periode meting/3(fs)
  Periode meting/1(pulses) -> Periode/1
  In/1 -> NOT/1, Edge Detector1/1
  Gain/1 -> Gain4/1
  Constant/1 -> Periode meting/4(reset)
  OR/1 -> Periode meting/1(speedPulse)
  Edge Detector1/1 -> OR/1
  Edge Detector2/1 -> OR/2
  NOT/1 -> Edge Detector2/1
  Gain4/1 -> Out/1

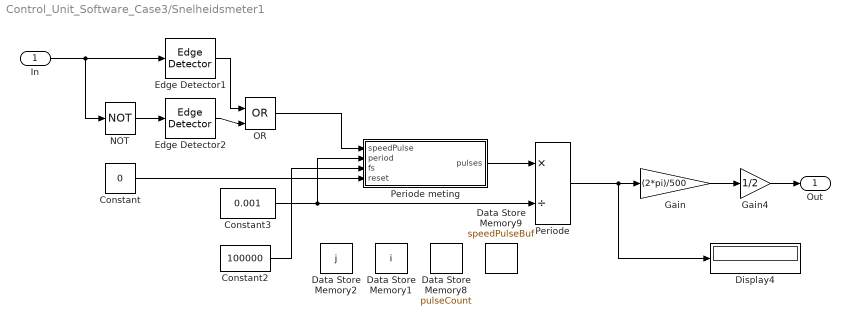
== system Control_Unit_Software_Case3/Snelheidsmeter1 ==
  In : Inport
  Constant : Constant  Value=0
  Constant2 : Constant  Value=100000
  Constant3 : Constant  Value=0.001
  Data Store Memory1 : DataStoreMemory  DataStoreName=i  ReadBeforeWriteMsg=warning  WriteAfterWriteMsg=warning  WriteAfterReadMsg=warning  InitialValue=1  ShowAdditionalParam=off  OutDataTypeStr=uint32
  Data Store Memory2 : DataStoreMemory  DataStoreName=j  ReadBeforeWriteMsg=warning  WriteAfterWriteMsg=warning  WriteAfterReadMsg=warning  InitialValue=2  ShowAdditionalParam=off  OutDataTypeStr=uint32
  Data Store Memory8 : DataStoreMemory  DataStoreName=pulseCount  ReadBeforeWriteMsg=warning  WriteAfterWriteMsg=warning  WriteAfterReadMsg=warning  ShowAdditionalParam=off  OutDataTypeStr=uint32
  Data Store Memory9 : DataStoreMemory  DataStoreName=speedPulseBuf  ReadBeforeWriteMsg=warning  WriteAfterWriteMsg=warning  WriteAfterReadMsg=warning  ShowAdditionalParam=off  OutDataTypeStr=uint8  Dimensions=10001
  Display4 : Display
  Edge Detector1 : dspswit3/Edge Detector  InputProcessing=Columns as channels (frame based)
      settings: SourceProductName=DSP System Toolbox  SourceProductBaseCode=DS
  Edge Detector2 : dspswit3/Edge Detector  InputProcessing=Columns as channels (frame based)
      settings: SourceProductName=DSP System Toolbox  SourceProductBaseCode=DS
  Gain : Gain  Gain=(2*pi)/500
  Gain4 : Gain  Gain=1/2
  NOT : Logic  Operator=NOT  IconShape=distinctive  AllPortsSameDT=off  OutDataTypeStr=boolean
  OR : Logic  Operator=OR  IconShape=distinctive  AllPortsSameDT=off  OutDataTypeStr=boolean
  Periode : Product  Inputs=*/
  Periode meting : MATLAB Function  TreatAsAtomicUnit=on
  Out : Outport
  wires:
  Constant3/1 -> Periode/2, Periode meting/2(period)
  Periode/1 -> Gain/1, Display4/1
  Constant2/1 -> Periode meting/3(fs)
  Periode meting/1(pulses) -> Periode/1
  In/1 -> NOT/1, Edge Detector1/1
  Gain/1 -> Gain4/1
  Constant/1 -> Periode meting/4(reset)
  OR/1 -> Periode meting/1(speedPulse)
  Edge Detector1/1 -> OR/1
  Edge Detector2/1 -> OR/2
  NOT/1 -> Edge Detector2/1
  Gain4/1 -> Out/1

== system Control_Unit_Software_Case3/Stroom links ==
  Demux : Demux  Tag=STV Demux  Outputs=1
  FromWs : FromWorkspace  Tag=STV FromWs  VariableName=tuvar  SampleTime=0
      SigBuilderData=|
      | common.afterFinalStr = 'Extrapolate'
      | common.sampleTime = 0
      | dataSet.timeRange = [0 10]
      | dataSet.name = 'Group 1'
      | sbobj.Groups.Name = 'Group 1'
      | sbobj.Groups.Signals.Name = 'Stroom links'
      | sbobj.Groups.Signals.XData = [0 1 1.5 2 7 10]
      | sbobj.Groups.Signals.YData = [0 0 30 0 0 0]
  Stroom links : Outport  Tag=STV Outport
  wires:
  Demux/1 -> Stroom links/1
  FromWs/1 -> Demux/1

== system Control_Unit_Software_Case3/Stroom rechts ==
  Demux : Demux  Tag=STV Demux  Outputs=1
  FromWs : FromWorkspace  Tag=STV FromWs  VariableName=tuvar  SampleTime=0
      SigBuilderData=|
      | common.afterFinalStr = 'Extrapolate'
      | common.sampleTime = 0
      | dataSet.timeRange = [0 10]
      | dataSet.name = 'Group 1'
      | sbobj.Groups.Name = 'Group 1'
      | sbobj.Groups.Signals.Name = 'Stroom rechts'
      | sbobj.Groups.Signals.XData = [0 2 2.5 3 7 10]
      | sbobj.Groups.Signals.YData = [0 0 30 0 0 0]
  Stroom rechts : Outport  Tag=STV Outport
  wires:
  Demux/1 -> Stroom rechts/1
  FromWs/1 -> Demux/1

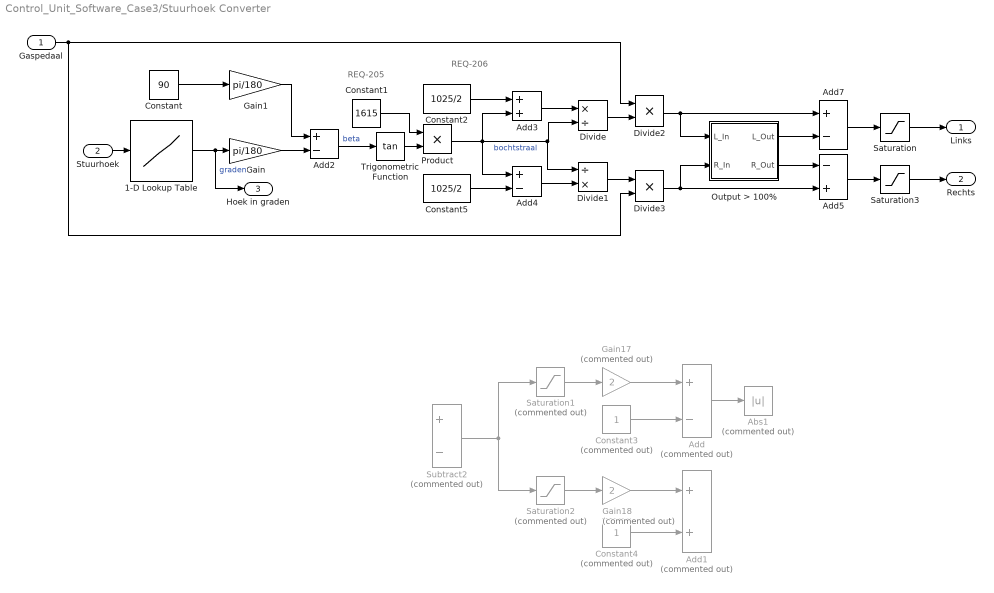
== system Control_Unit_Software_Case3/Stuurhoek Converter ==
  note: REQ-205
  note: REQ-206
  "Gaspedaal " : Inport
  Stuurhoek : Inport  Port=2
  1-D Lookup Table : Lookup_n-D  NumberOfTableDimensions=1  BreakpointsForDimension1=[0 0.5 1]  Table=[-30 0 30]  InternalRulePriority=Speed  RndMeth=Simplest  InputSameDT=on
  Abs1 : Abs  Commented=on
  Add : Sum  Commented=on  Inputs=+-
  Add1 : Sum  Commented=on
  Add2 : Sum  Inputs=+-
  Add3 : Sum
  Add4 : Sum  Inputs=+-
  Add5 : Sum  Inputs=-+
  Add7 : Sum  Inputs=+-
  Constant : Constant  Value=90
  Constant1 : Constant  Value=1615
  Constant2 : Constant  Value=1025/2
  Constant3 : Constant  Commented=on
  Constant4 : Constant  Commented=on
  Constant5 : Constant  Value=1025/2
  Divide : Product  Inputs=*/
  Divide1 : Product  Inputs=/*
  Divide2 : Product  Inputs=**
  Divide3 : Product  Inputs=**
  Gain : Gain  Gain=pi/180
  Gain1 : Gain  Gain=pi/180
  Gain17 : Gain  Commented=on  Gain=2
  Gain18 : Gain  Commented=on  Gain=2
  Output > 100% : Subsystem
  Product : Product
  Saturation : Saturate  UpperLimit=1  LowerLimit=0
  Saturation1 : Saturate  Commented=on  LowerLimit=0
  Saturation2 : Saturate  Commented=on  UpperLimit=0
  Saturation3 : Saturate  UpperLimit=1  LowerLimit=0
  Subtract2 : Sum  Commented=on  Inputs=+-
  Trigonometric Function : Trigonometry  Operator=tan
  Links : Outport
  Rechts : Outport  Port=2
  Hoek in graden : Outport  Port=3
  wires:
  Saturation1/1 -> Gain17/1
  Subtract2/1 -> Saturation2/1, Saturation1/1
  Gain18/1 -> Add1/1
  Add/1 -> Abs1/1
  Saturation2/1 -> Gain18/1
  Gain17/1 -> Add/1
  Constant4/1 -> Add1/2
  Constant3/1 -> Add/2
  1-D Lookup Table/1 -> Hoek in graden/1, Gain/1  "graden"
  Constant/1 -> Gain1/1
  Add2/1 -> Trigonometric Function/1  "beta"
  Constant1/1 -> Product/1
  Trigonometric Function/1 -> Product/2
  Product/1 -> Divide1/1, Divide/2, Add4/1, Add3/2  "bochtstraal"
  Constant2/1 -> Add3/1
  Add3/1 -> Divide/1
  Constant5/1 -> Add4/2
  Add4/1 -> Divide1/2
  Divide1/1 -> Divide3/1
  Divide/1 -> Divide2/2
  "Gaspedaal "/1 -> Divide2/1, Divide3/2
  Divide2/1 -> Add7/1, Output > 100%/1(L_In)
  Divide3/1 -> Output > 100%/2(R_In), Add5/2
  Stuurhoek/1 -> 1-D Lookup Table/1
  Gain/1 -> Add2/2
  Gain1/1 -> Add2/1
  Add7/1 -> Saturation/1
  Add5/1 -> Saturation3/1
  Output > 100%/1(L_Out) -> Add7/2
  Output > 100%/2(R_Out) -> Add5/1
  Saturation/1 -> Links/1
  Saturation3/1 -> Rechts/1

== system Control_Unit_Software_Case3/Temperatuur links ==
  Demux : Demux  Tag=STV Demux  Outputs=1
  FromWs : FromWorkspace  Tag=STV FromWs  VariableName=tuvar  SampleTime=0
      SigBuilderData=|
      | common.afterFinalStr = 'Extrapolate'
      | common.sampleTime = 0
      | dataSet.timeRange = [0 15]
      | dataSet.name = 'Group 1'
      | sbobj.Groups.Name = 'Group 1'
      | sbobj.Groups.Signals.Name = 'Temperatuur links'
      | sbobj.Groups.Signals.XData = [0 5 5.5 6 7 10 11 11.65 13 13.5 14.2 15]
      | sbobj.Groups.Signals.YData = [0 0 150 0 0 0 119 0 0 150 0 0]
      | sbobj.Groups.TimeRange = [0 15]
  Temperatuur links : Outport  Tag=STV Outport
  wires:
  Demux/1 -> Temperatuur links/1
  FromWs/1 -> Demux/1

== system Control_Unit_Software_Case3/Temperatuur rechts ==
  Demux : Demux  Tag=STV Demux  Outputs=1
  FromWs : FromWorkspace  Tag=STV FromWs  VariableName=tuvar  SampleTime=0
      SigBuilderData=|
      | common.afterFinalStr = 'Extrapolate'
      | common.sampleTime = 0
      | dataSet.timeRange = [0 10]
      | dataSet.name = 'Group 1'
      | sbobj.Groups.Name = 'Group 1'
      | sbobj.Groups.Signals.Name = 'Temperatuur rechts'
      | sbobj.Groups.Signals.XData = [0 8 8.5 9 10]
      | sbobj.Groups.Signals.YData = [0 0 150 0 0]
  Temperatuur rechts : Outport  Tag=STV Outport
  wires:
  Demux/1 -> Temperatuur rechts/1
  FromWs/1 -> Demux/1

== system Control_Unit_Software_Case3/Vooruit // achteruit ==
  Demux : Demux  Tag=STV Demux  Outputs=1
  FromWs : FromWorkspace  Tag=STV FromWs  VariableName=tuvar  SampleTime=0
      SigBuilderData=|
      | common.afterFinalStr = 'Extrapolate'
      | common.sampleTime = 0
      | dataSet.timeRange = [0 10]
      | dataSet.name = 'Group 1'
      | sbobj.Groups.Name = 'Group 1'
      | sbobj.Groups.Signals.Name = 'Vooruit/achteruit'
      | sbobj.Groups.Signals.XData = [0 0.5 0.5 10]
      | sbobj.Groups.Signals.YData = [1 1 0 0]
  Vooruit/achteruit : Outport  Tag=STV Outport
  wires:
  Demux/1 -> Vooruit/achteruit/1
  FromWs/1 -> Demux/1

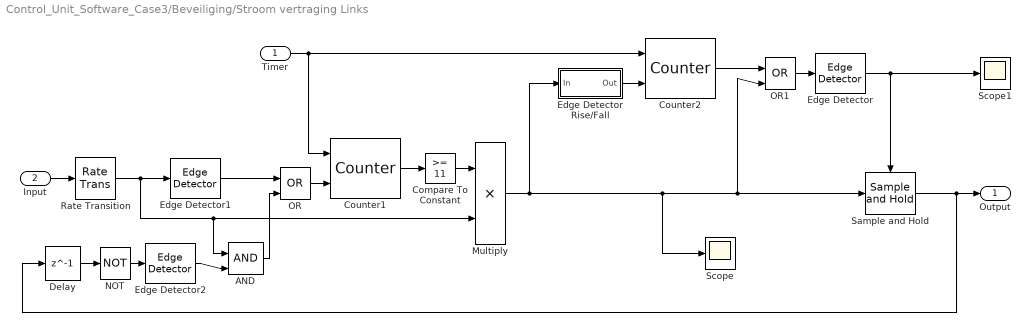
== system Control_Unit_Software_Case3/Beveiliging/Stroom vertraging Links ==
  Timer : Inport
  Input : Inport  Port=2
  AND : Logic  IconShape=distinctive  AllPortsSameDT=off  OutDataTypeStr=boolean
  Compare To Constant : simulink/Logic and Bit Operations/Compare To Constant  relop=>=  const=11  OutDataTypeStr=boolean
  Counter1 : dspswit3/Counter  Direction=Up  CountEvent=Rising edge  CounterSize=32 bits  MaxCount=20  InitialCount=0  Output=Count  HitValue=20  ResetInput=on  SamplesPerFrame=1  Ts=1  CntDtype=double  HitDtype=Logical
  Counter2 : dspswit3/Counter  Direction=Up  CountEvent=Rising edge  CounterSize=User defined  MaxCount=300  InitialCount=0  Output=Hit  HitValue=300  ResetInput=on  SamplesPerFrame=1  Ts=1  CntDtype=double  HitDtype=Logical
  Delay : Delay  DelayLength=1
  Edge Detector : dspswit3/Edge Detector  InputProcessing=Columns as channels (frame based)
      settings: SourceProductName=DSP System Toolbox  SourceProductBaseCode=DS
  Edge Detector1 : dspswit3/Edge Detector  InputProcessing=Columns as channels (frame based)
      settings: SourceProductName=DSP System Toolbox  SourceProductBaseCode=DS
  Edge Detector2 : dspswit3/Edge Detector  InputProcessing=Columns as channels (frame based)
      settings: SourceProductName=DSP System Toolbox  SourceProductBaseCode=DS
  Edge Detector Rise/Fall : Subsystem
  Multiply : Product
  NOT : Logic  Operator=NOT  IconShape=distinctive  AllPortsSameDT=off  OutDataTypeStr=boolean
  OR : Logic  Operator=OR  IconShape=distinctive  AllPortsSameDT=off  OutDataTypeStr=boolean
  OR1 : Logic  Operator=OR  IconShape=distinctive  AllPortsSameDT=off  OutDataTypeStr=boolean
  Rate Transition : RateTransition  OutPortSampleTime=1/1000
  Sample and Hold : dspsigops/Sample and Hold  trig=Rising edge  initCond=0  latchinput=off
  Scope : Scope
  Scope1 : Scope
  Output : Outport
  wires:
  Timer/1 -> Counter2/1, Counter1/1
  Sample and Hold/1 -> Output/1, Delay/1
  OR1/1 -> Edge Detector/1
  Edge Detector/1 -> Scope1/1, Sample and Hold/Trigger
  Counter2/1 -> OR1/1
  Multiply/1 -> Edge Detector Rise/Fall/1(In), OR1/2, Sample and Hold/1, Scope/1
  Edge Detector Rise/Fall/1(Out) -> Counter2/2
  Counter1/1 -> Compare To Constant/1
  Input/1 -> Rate Transition/1
  Rate Transition/1 -> Multiply/2, AND/1, Edge Detector1/1
  NOT/1 -> Edge Detector2/1
  Edge Detector2/1 -> AND/2
  AND/1 -> OR/2
  OR/1 -> Counter1/2
  Edge Detector1/1 -> OR/1
  Delay/1 -> NOT/1
  Compare To Constant/1 -> Multiply/1

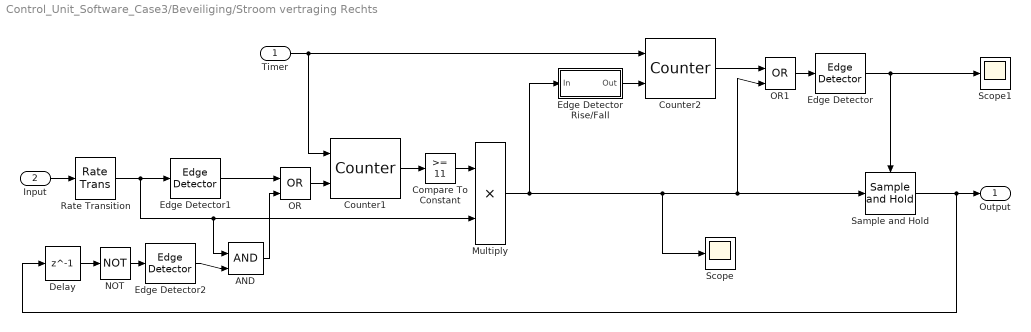
== system Control_Unit_Software_Case3/Beveiliging/Stroom vertraging Rechts ==
  Timer : Inport
  Input : Inport  Port=2
  AND : Logic  IconShape=distinctive  AllPortsSameDT=off  OutDataTypeStr=boolean
  Compare To Constant : simulink/Logic and Bit Operations/Compare To Constant  relop=>=  const=11  OutDataTypeStr=boolean
  Counter1 : dspswit3/Counter  Direction=Up  CountEvent=Rising edge  CounterSize=32 bits  MaxCount=20  InitialCount=0  Output=Count  HitValue=20  ResetInput=on  SamplesPerFrame=1  Ts=1  CntDtype=double  HitDtype=Logical
  Counter2 : dspswit3/Counter  Direction=Up  CountEvent=Rising edge  CounterSize=User defined  MaxCount=300  InitialCount=0  Output=Hit  HitValue=300  ResetInput=on  SamplesPerFrame=1  Ts=1  CntDtype=double  HitDtype=Logical
  Delay : Delay  DelayLength=1
  Edge Detector : dspswit3/Edge Detector  InputProcessing=Columns as channels (frame based)
      settings: SourceProductName=DSP System Toolbox  SourceProductBaseCode=DS
  Edge Detector1 : dspswit3/Edge Detector  InputProcessing=Columns as channels (frame based)
      settings: SourceProductName=DSP System Toolbox  SourceProductBaseCode=DS
  Edge Detector2 : dspswit3/Edge Detector  InputProcessing=Columns as channels (frame based)
      settings: SourceProductName=DSP System Toolbox  SourceProductBaseCode=DS
  Edge Detector Rise/Fall : Subsystem
  Multiply : Product
  NOT : Logic  Operator=NOT  IconShape=distinctive  AllPortsSameDT=off  OutDataTypeStr=boolean
  OR : Logic  Operator=OR  IconShape=distinctive  AllPortsSameDT=off  OutDataTypeStr=boolean
  OR1 : Logic  Operator=OR  IconShape=distinctive  AllPortsSameDT=off  OutDataTypeStr=boolean
  Rate Transition : RateTransition  OutPortSampleTime=1/1000
  Sample and Hold : dspsigops/Sample and Hold  trig=Rising edge  initCond=0  latchinput=off
  Scope : Scope
  Scope1 : Scope
  Output : Outport
  wires:
  Timer/1 -> Counter2/1, Counter1/1
  Sample and Hold/1 -> Output/1, Delay/1
  OR1/1 -> Edge Detector/1
  Edge Detector/1 -> Scope1/1, Sample and Hold/Trigger
  Counter2/1 -> OR1/1
  Multiply/1 -> Edge Detector Rise/Fall/1(In), OR1/2, Sample and Hold/1, Scope/1
  Edge Detector Rise/Fall/1(Out) -> Counter2/2
  Counter1/1 -> Compare To Constant/1
  Input/1 -> Rate Transition/1
  Rate Transition/1 -> Multiply/2, AND/1, Edge Detector1/1
  NOT/1 -> Edge Detector2/1
  Edge Detector2/1 -> AND/2
  AND/1 -> OR/2
  OR/1 -> Counter1/2
  Edge Detector1/1 -> OR/1
  Delay/1 -> NOT/1
  Compare To Constant/1 -> Multiply/1

== system Control_Unit_Software_Case3/Beveiliging/Temperatuur beperking ==
  T1 : Inport
  T2 : Inport  Port=2
  Constant5 : Constant
  Divide : Product  Inputs=*/
  Max : MinMax  Function=max  Inputs=2
  Range : Constant  Value=40
  Saturation : Saturate  UpperLimit=inf  LowerLimit=0
  Subtract : Sum  Inputs=+-
  Subtract1 : Sum  Inputs=+-
  Threshold : Constant  Value=80
  Out : Outport
  wires:
  Subtract/1 -> Saturation/1
  Divide/1 -> Subtract1/2
  Constant5/1 -> Subtract1/1
  Threshold/1 -> Subtract/2
  Max/1 -> Subtract/1
  T2/1 -> Max/2
  Range/1 -> Divide/2
  Saturation/1 -> Divide/1
  Subtract1/1 -> Out/1
  T1/1 -> Max/1

== system Control_Unit_Software_Case3/Beveiliging/Temperatuur vertraging Links ==
  Timer : Inport
  Input : Inport  Port=2
  Counter2 : dspswit3/Counter  Direction=Up  CountEvent=Rising edge  CounterSize=User defined  MaxCount=300  InitialCount=0  Output=Hit  HitValue=300  ResetInput=on  SamplesPerFrame=1  Ts=1  CntDtype=double  HitDtype=Logical
  Edge Detector : dspswit3/Edge Detector  InputProcessing=Columns as channels (frame based)
      settings: SourceProductName=DSP System Toolbox  SourceProductBaseCode=DS
  Edge Detector Rise/Fall : Subsystem
  OR1 : Logic  Operator=OR  IconShape=distinctive  AllPortsSameDT=off  OutDataTypeStr=boolean
  Sample and Hold : dspsigops/Sample and Hold  trig=Rising edge  initCond=0  latchinput=off
  Scope : Scope
  Scope1 : Scope
  Output : Outport
  wires:
  Timer/1 -> Counter2/1
  Sample and Hold/1 -> Output/1
  OR1/1 -> Edge Detector/1
  Edge Detector/1 -> Scope1/1, Sample and Hold/Trigger
  Counter2/1 -> OR1/1
  Input/1 -> Scope/1, OR1/2, Sample and Hold/1, Edge Detector Rise/Fall/1(In)
  Edge Detector Rise/Fall/1(Out) -> Counter2/2
